simulink model "Test_anode_system"  (R2023a)
settings: Solver=VariableStepAuto  StartTime=0.0  StopTime=100  RelTol=1e-3
libraries: nesl_utility x13, fl_lib x8
settings Model: Creator=debjani.ghosh  LastModifiedBy=debjani.ghosh

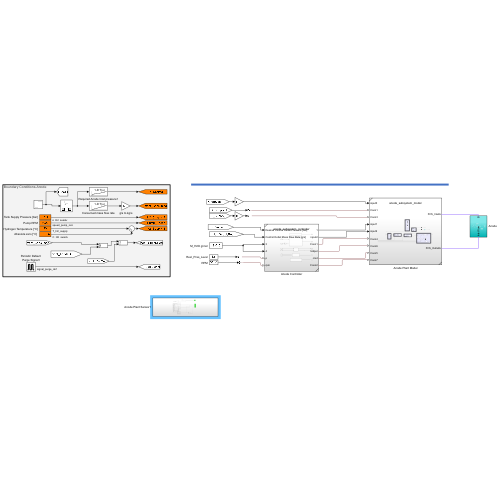
[thumbnail: Simulink's stored preview of the top-level diagram]
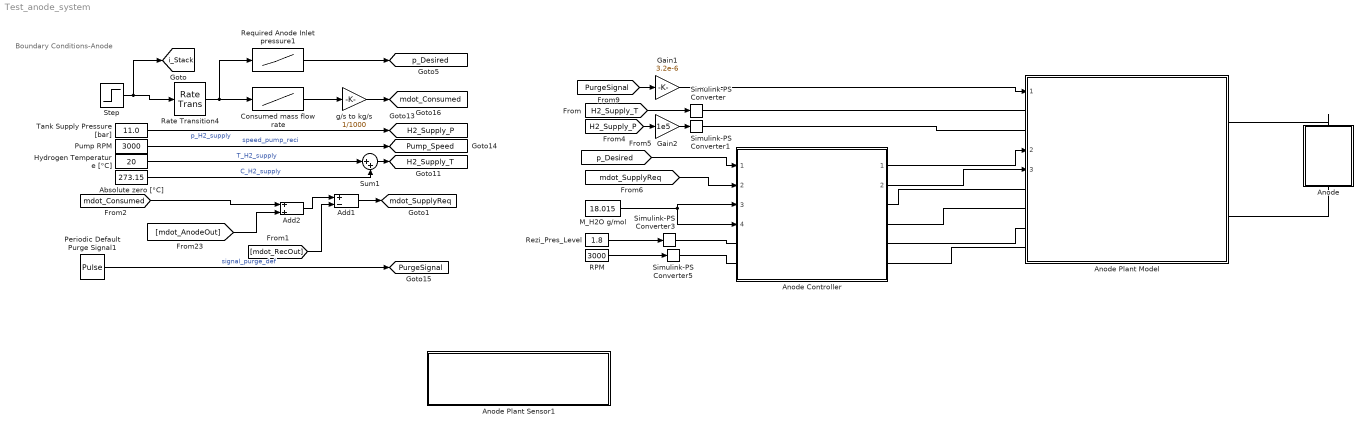
== system Test_anode_system ==
  note: Boundary Conditions-Anode
  "Absolute zero [°C] " : Constant  Value=273.15
  Add1 : Sum  Inputs=+-
  Add2 : Sum
  Anode : Subsystem  Tag=PublishSubsystem
  Anode Controller : Subsystem  ReferencedSubsystem=anode_subsystem_controller
  Anode Plant Model : Subsystem  ReferencedSubsystem=anode_subsystem_model
      settings: PortSchema="{\"entries\":[{\"content\":{\"sides\":[{\"content\":{\"connectorIds\":[\"In1\",\"LConn1\",\"LConn2\",\"In2\",\"In3\",\"LConn3\",\"LConn4\",\"LConn5\",\"LConn6\"]},\"type\":\"ConnectorPlacement.EquallySpacedRectSide\",\"uuid\":\"6d276737-1cfb-43f0-89a6-ca57f89f04f9\"},{\"content\":{\"connectorIds\":[\"RConn1\",\"RConn2\"],\"side\":\"RIGHT\"},\"type\":\"ConnectorPlacement.EquallySpacedRectSide\",\"uuid\":\"f7ce7b2b-f458-4a7d-a84b-f12d4a9a3d73\"},{\"content\":{\"side\":\"TOP\"},\"type\":\"ConnectorPlacement.EquallySpacedRectSide\",\"uuid\":\"f2759a84-f209-4626-aa5e-b52256180764\"}]},\"type\":\"ConnectorPlacement.EquallySpacedConnector\",\"uuid\":\"a55dce8e-c3c8-40fa-9a6a-dcd78737938e\"}],\"packageUris\":[\"http://schema.mathworks.com/mf0/Connector/R2020b\"],\"version\":\"1.0\"}"
  Anode Plant Sensor1 : Subsystem
  Consumed mass flow rate : Lookup_n-D  NumberOfTableDimensions=1  BreakpointsForDimension1=[0;20;100;200;300;400;500;600]  Table=[0;0.1;0.5;1;1.5;2;2.5;3]  InternalRulePriority=Speed  RndMeth=Simplest
  Gain1 : Gain  Gain=3.2e-6
  Gain2 : Gain  Gain=1e5
  Hydrogen Temperature [°C] : Constant  Value=20
  M_H2O g/mol : Constant  Value=18.015
  Periodic Default Purge Signal1 : DiscretePulseGenerator  PulseType=Time based  Period=3  PulseWidth=5
  Pump RPM : Constant  Value=3000
  RPM : Constant  Value=3000
  Rate Transition4 : RateTransition
  Required Anode Inlet pressure1 : Lookup_n-D  NumberOfTableDimensions=1  BreakpointsForDimension1=[0;20;100;200;300;400;500;600]  Table=[1;1.4;1.6;1.7;1.8;2;2.3;2.6]  InternalRulePriority=Speed  RndMeth=Simplest
  Rezi_Pres_Level : Constant  Value=1.8
  Simulink-PS Converter : nesl_utility/Simulink-PS Converter  PhysicalDomain=network_engine_domain  SubClassName=ps_input  LeftPortType=input  RightPortType=output  PseudoPeriodic=off  Frequencies=[]  NoiseDistribution=none  NoiseParameters=[]  Unit=K  AffineConversion=off  FilteringAndDerivatives=provide  SimscapeFilterOrder=1  InputFilterTimeConstant=0.001  UdotUserProvided=0
  Simulink-PS Converter1 : nesl_utility/Simulink-PS Converter  PhysicalDomain=network_engine_domain  SubClassName=ps_input  LeftPortType=input  RightPortType=output  PseudoPeriodic=off  Frequencies=[]  NoiseDistribution=none  NoiseParameters=[]  Unit=Pa  AffineConversion=off  FilteringAndDerivatives=provide  SimscapeFilterOrder=1  InputFilterTimeConstant=0.001  UdotUserProvided=0
  Simulink-PS Converter3 : nesl_utility/Simulink-PS Converter  PhysicalDomain=network_engine_domain  SubClassName=ps_input  LeftPortType=input  RightPortType=output  PseudoPeriodic=off  Frequencies=[]  NoiseDistribution=none  NoiseParameters=[]  Unit=1  AffineConversion=off  FilteringAndDerivatives=provide  SimscapeFilterOrder=1  InputFilterTimeConstant=0.001  UdotUserProvided=0
  Simulink-PS Converter5 : nesl_utility/Simulink-PS Converter  PhysicalDomain=network_engine_domain  SubClassName=ps_input  LeftPortType=input  RightPortType=output  PseudoPeriodic=off  Frequencies=[]  NoiseDistribution=none  NoiseParameters=[]  Unit=1  AffineConversion=off  FilteringAndDerivatives=provide  SimscapeFilterOrder=1  InputFilterTimeConstant=0.001  UdotUserProvided=0
  Step : Step  Time=50  Before=200  After=400  SampleTime=0
  Sum1 : Sum  Inputs=|++
  Tank Supply Pressure [bar] : Constant  Value=11.0
  g/s to kg/s : Gain  Gain=1/1000
  tag scope: H2_Supply_P=global, H2_Supply_T=global, Pump_Speed=global, PurgeSignal=global, i_Stack=global, mdot_Consumed=global, mdot_SupplyReq=global, p_Desired=global
  wires:
  Sum1/1 -> [H2_Supply_T]
  Gain1/1 -> Anode Plant Model/1
  [p_Desired] -> Anode Controller/1
  g/s to kg/s/1 -> [mdot_Consumed]
  [H2_Supply_T] -> Simulink-PS Converter/1
  "Absolute zero [°C] "/1 -> Sum1/2  "C_H2_supply"
  RPM/1 -> Simulink-PS Converter5/1
  Rezi_Pres_Level/1 -> Simulink-PS Converter3/1
  Periodic Default Purge Signal1/1 -> [PurgeSignal]  "signal_purge_def"
  Consumed mass flow rate/1 -> g/s to kg/s/1
  [PurgeSignal] -> Gain1/1
  [mdot_SupplyReq] -> Anode Controller/2
  [H2_Supply_P] -> Gain2/1
  Anode Controller/1 -> Anode Plant Model/2
  Gain2/1 -> Simulink-PS Converter1/1
  M_H2O g/mol/1 -> Anode Controller/3, Anode Controller/4
  Pump RPM/1 -> [Pump_Speed]  "speed_pump_reci"
  Rate Transition4/1 -> Required Anode Inlet pressure1/1, Consumed mass flow rate/1
  Required Anode Inlet pressure1/1 -> [p_Desired]
  Anode Controller/2 -> Anode Plant Model/3
  Tank Supply Pressure [bar]/1 -> [H2_Supply_P]  "p_H2_supply"
  Hydrogen Temperature [°C]/1 -> Sum1/1  "T_H2_supply"
  Step/1 -> [i_Stack], Rate Transition4/1
  [mdot_AnodeOut] -> Add2/2
  Add2/1 -> Add1/1
  [mdot_Consumed] -> Add2/1
  Add1/1 -> [mdot_SupplyReq]
  [mdot_RecOut] -> Add1/2
  connections:
  Simulink-PS Converter/RConn1 -- Anode Plant Model/LConn1
  Anode Plant Model/LConn6 -- Anode Controller/RConn4
  Anode Plant Model/LConn2 -- Simulink-PS Converter1/RConn1
  Anode Controller/RConn3 -- Anode Plant Model/LConn5
  Anode Controller/LConn1 -- Simulink-PS Converter3/RConn1
  Anode Controller/RConn2 -- Anode Plant Model/LConn4
  Anode Controller/RConn1 -- Anode Plant Model/LConn3
  Simulink-PS Converter5/RConn1 -- Anode Controller/LConn2
  Anode/LConn1 -- Anode Plant Model/RConn1
  Anode/RConn1 -- Anode Plant Model/RConn2

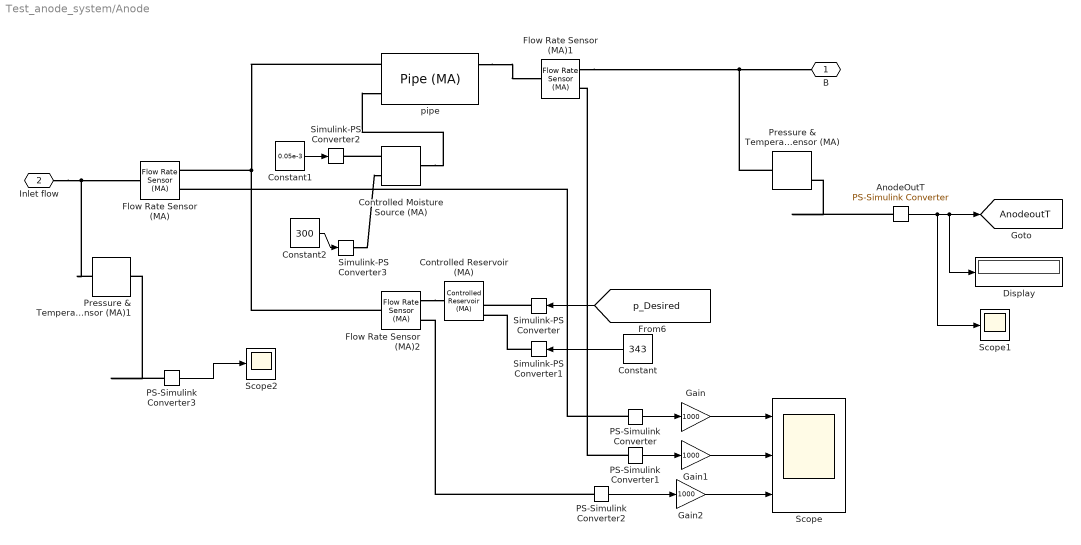
== system Test_anode_system/Anode ==
  AnodeOutT : nesl_utility/PS-Simulink Converter  PhysicalDomain=network_engine_domain  SubClassName=ps_output  LeftPortType=input  RightPortType=output  PseudoPeriodic=off  Frequencies=[]  VectorFormat=inherit  Unit=inherit  AffineConversion=off
  Constant : Constant  Value=343
  Constant1 : Constant  Value=0.05e-3
  Constant2 : Constant  Value=300
  Controlled Moisture Source (MA) : fl_lib/Moist Air/Sources/Moisture & Trace Gas Sources/Controlled Moisture Source (MA)  moisture_source_spec=foundation.enum.moisture_source_spec.vapor  Phi_S_specify=off  Phi_S_priority=None  Phi_S=0 kW  Phi_S_nominal_specify=off  Phi_S_nominal_unit=kW  Phi_S_nominal_value=1  mdot_w_S_specify=off  mdot_w_S_priority=None  mdot_w_S=0 kg/s  mdot_w_S_nominal_specify=off  mdot_w_S_nominal_unit=kg/s  mdot_w_S_nominal_value=1
      settings: InternalSimscapePortConfiguration="{\"Bottom\":[],\"Left\":[{\"id\":\"S\",\"label\":\"S\",\"type\":\"foundation.moist_air.moist_air_source\"}],\"Right\":[{\"id\":\"M\",\"label\":\"M\",\"type\":\"input\"},{\"id\":\"T\",\"label\":\"T\",\"type\":\"input\"}],\"Top\":[]}"
  Controlled Reservoir (MA) : fl_lib/Moist Air/Elements/Controlled Reservoir (MA)  moisture_spec=foundation.enum.moistureSpec.RelativeHumidity  trace_gas_spec=foundation.enum.trace_gas_spec.mass_fraction  RH_ws=1  area_A=0.01 m^2  input_error_spec=foundation.enum.input_range_error.warn
      settings: InternalSimscapePortConfiguration="{\"Bottom\":[],\"Left\":[{\"id\":\"A\",\"label\":\"A\",\"type\":\"foundation.moist_air.moist_air\"}],\"Right\":[{\"id\":\"T\",\"label\":\"T\",\"type\":\"input\"},{\"id\":\"P\",\"label\":\"P\",\"type\":\"input\"},{\"id\":\"W\",\"label\":\"W\",\"type\":\"input\"},{\"id\":\"G\",\"label\":\"G\",\"type\":\"input\"}],\"Top\":[]}"
  Display : Display
  Flow Rate Sensor (MA) : fl_lib/Moist Air/Sensors/Flow Rate Sensor (MA)  mass_flow_measure=true  volumetric_flow_measure=false  volumetric_flow_conditions=foundation.enum.volumetric_flow_conditions.actual  p_std=0.101325 MPa  T_std=20 degC  RH_std=0.65  energy_flow_measure=false  vapor_flow_measure=false  gas_flow_measure=false
      settings: InternalSimscapePortConfiguration="{\"Bottom\":[],\"Left\":[{\"id\":\"A\",\"label\":\"A\",\"type\":\"foundation.moist_air.moist_air\"}],\"Right\":[{\"id\":\"B\",\"label\":\"B\",\"type\":\"foundation.moist_air.moist_air\"},{\"id\":\"M\",\"label\":\"M\",\"type\":\"output\"}],\"Top\":[]}"
  Flow Rate Sensor (MA)1 : fl_lib/Moist Air/Sensors/Flow Rate Sensor (MA)  mass_flow_measure=true  volumetric_flow_measure=false  volumetric_flow_conditions=foundation.enum.volumetric_flow_conditions.actual  p_std=0.101325 MPa  T_std=20 degC  RH_std=0.65  energy_flow_measure=false  vapor_flow_measure=false  gas_flow_measure=false
      settings: InternalSimscapePortConfiguration="{\"Bottom\":[],\"Left\":[{\"id\":\"A\",\"label\":\"A\",\"type\":\"foundation.moist_air.moist_air\"}],\"Right\":[{\"id\":\"B\",\"label\":\"B\",\"type\":\"foundation.moist_air.moist_air\"},{\"id\":\"M\",\"label\":\"M\",\"type\":\"output\"}],\"Top\":[]}"
  Flow Rate Sensor (MA)2 : fl_lib/Moist Air/Sensors/Flow Rate Sensor (MA)  mass_flow_measure=true  volumetric_flow_measure=false  volumetric_flow_conditions=foundation.enum.volumetric_flow_conditions.actual  p_std=0.101325 MPa  T_std=20 degC  RH_std=0.65  energy_flow_measure=false  vapor_flow_measure=false  gas_flow_measure=false
      settings: InternalSimscapePortConfiguration="{\"Bottom\":[],\"Left\":[{\"id\":\"A\",\"label\":\"A\",\"type\":\"foundation.moist_air.moist_air\"}],\"Right\":[{\"id\":\"B\",\"label\":\"B\",\"type\":\"foundation.moist_air.moist_air\"},{\"id\":\"M\",\"label\":\"M\",\"type\":\"output\"}],\"Top\":[]}"
  Gain : Gain  Gain=1000
  Gain1 : Gain  Gain=1000
  Gain2 : Gain  Gain=1000
  PS-Simulink Converter{,1..3} (4 alike) : nesl_utility/PS-Simulink Converter  PhysicalDomain=network_engine_domain  SubClassName=ps_output  LeftPortType=input  RightPortType=output  PseudoPeriodic=off  Frequencies=[]  VectorFormat=inherit  Unit=inherit  AffineConversion=off
  Pressure & Temperature Sensor (MA) : fl_lib/Moist Air/Sensors/Pressure & Temperature Sensor (MA)  reference=foundation.enum.MeasurementReference.absolute  pressure=true  pressure_spec=foundation.enum.PressureMeasementSpec.Absolute  temperature=true
      settings: InternalSimscapePortConfiguration="{\"Bottom\":[{\"id\":\"T\",\"label\":\"T\",\"type\":\"output\"}],\"Left\":[{\"id\":\"A\",\"label\":\"A\",\"type\":\"foundation.moist_air.moist_air\"}],\"Right\":[{\"id\":\"Pa\",\"label\":\"Pa\",\"type\":\"output\"}],\"Top\":[]}"
  Pressure & Temperature Sensor (MA)1 : fl_lib/Moist Air/Sensors/Pressure & Temperature Sensor (MA)  reference=foundation.enum.MeasurementReference.absolute  pressure=false  pressure_spec=foundation.enum.PressureMeasementSpec.Absolute  temperature=true
      settings: InternalSimscapePortConfiguration="{\"Bottom\":[{\"id\":\"T\",\"label\":\"T\",\"type\":\"output\"}],\"Left\":[{\"id\":\"A\",\"label\":\"A\",\"type\":\"foundation.moist_air.moist_air\"}],\"Right\":[],\"Top\":[]}"
  Scope : Scope  NumInputPorts=3
  Scope1 : Scope
  Scope2 : Scope
  Simulink-PS Converter : nesl_utility/Simulink-PS Converter  PhysicalDomain=network_engine_domain  SubClassName=ps_input  LeftPortType=input  RightPortType=output  PseudoPeriodic=off  Frequencies=[]  NoiseDistribution=none  NoiseParameters=[]  Unit=bar  AffineConversion=off  FilteringAndDerivatives=provide  SimscapeFilterOrder=1  InputFilterTimeConstant=0.001  UdotUserProvided=0
  Simulink-PS Converter1 : nesl_utility/Simulink-PS Converter  PhysicalDomain=network_engine_domain  SubClassName=ps_input  LeftPortType=input  RightPortType=output  PseudoPeriodic=off  Frequencies=[]  NoiseDistribution=none  NoiseParameters=[]  Unit=K  AffineConversion=off  FilteringAndDerivatives=provide  SimscapeFilterOrder=1  InputFilterTimeConstant=0.001  UdotUserProvided=0
  Simulink-PS Converter2 : nesl_utility/Simulink-PS Converter  PhysicalDomain=network_engine_domain  SubClassName=ps_input  LeftPortType=input  RightPortType=output  PseudoPeriodic=off  Frequencies=[]  NoiseDistribution=none  NoiseParameters=[]  Unit=1  AffineConversion=off  FilteringAndDerivatives=provide  SimscapeFilterOrder=1  InputFilterTimeConstant=0.001  UdotUserProvided=0
  Simulink-PS Converter3 : nesl_utility/Simulink-PS Converter  PhysicalDomain=network_engine_domain  SubClassName=ps_input  LeftPortType=input  RightPortType=output  PseudoPeriodic=off  Frequencies=[]  NoiseDistribution=none  NoiseParameters=[]  Unit=1  AffineConversion=off  FilteringAndDerivatives=provide  SimscapeFilterOrder=1  InputFilterTimeConstant=0.001  UdotUserProvided=0
  pipe : fl_lib/Moist Air/Elements/Pipe (MA)  length=0.25 m  area=pi*0.05^2/4 m^2  Dh=0.05 m  length_add=0.1 m  roughness=15e-6 m  Re_lam=2000  Re_tur=4000  shape_factor=64  Nu_lam=3.66  wall_condensation=simscape.enum.onoff.off  RH_ws=1  time_constant=1e-3 s  moisture_trace_gas_source=foundation.enum.moisture_trace_gas_source.controlled  moisture_source_spec=foundation.enum.moisture_source_spec.vapor  moisture_mass_flow=0 kg/s  moisture_temperature_spec=foundation.enum.temperature_spec.atmospheric  moisture_temperature=293.15 K  trace_gas_mass_flow=0 kg/s  trace_gas_temperature_spec=foundation.enum.temperature_spec.atmospheric  trace_gas_temperature=293.15 K  p_I_specify=on  p_I_priority=High  p_I=env_p MPa  p_I_nominal_specify=off  p_I_nominal_unit=MPa  p_I_nominal_value=1  T_I_specify=on  T_I_priority=High  T_I=env_T degC  T_I_nominal_specify=off  T_I_nominal_unit=K  T_I_nominal_value=1  RH_I_specify=off  RH_I_priority=High  RH_I=0  RH_I_nominal_specify=off  RH_I_nominal_unit=1  RH_I_nominal_value=1  x_w_I_specify=off  x_w_I_priority=None  x_w_I=0  x_w_I_nominal_specify=off  x_w_I_nominal_unit=1  x_w_I_nominal_value=1  y_w_I_specify=off  y_w_I_priority=None  y_w_I=0  y_w_I_nominal_specify=off  y_w_I_nominal_unit=1  y_w_I_nominal_value=1  HR_I_specify=off  HR_I_priority=None  HR_I=0  HR_I_nominal_specify=off  HR_I_nominal_unit=1  HR_I_nominal_value=1  x_g_I_specify=on  x_g_I_priority=None  x_g_I=0  x_g_I_nominal_specify=off  x_g_I_nominal_unit=1  x_g_I_nominal_value=1  y_g_I_specify=on  y_g_I_priority=High  y_g_I=tank_yH2  y_g_I_nominal_specify=off  y_g_I_nominal_unit=1  y_g_I_nominal_value=1
      settings: InternalSimscapePortConfiguration="{\"Bottom\":[],\"Left\":[{\"id\":\"A\",\"label\":\"A\",\"type\":\"foundation.moist_air.moist_air\"},{\"id\":\"H\",\"label\":\"H\",\"type\":\"foundation.thermal.thermal\"},{\"id\":\"S\",\"label\":\"S\",\"type\":\"foundation.moist_air.moist_air_source\"}],\"Right\":[{\"id\":\"B\",\"label\":\"B\",\"type\":\"foundation.moist_air.moist_air\"},{\"id\":\"W\",\"label\":\"W\",\"type\":\"output\"},{\"id\":\"F\",\"label\":\"F\",\"type\":\"output\"}],\"Top\":[]}"
  B : PMIOPort  Side=Left
  Inlet flow : PMIOPort  Port=2  Side=Right
  tag scope: AnodeoutT=global
  wires:
  [p_Desired] -> Simulink-PS Converter/1
  Constant/1 -> Simulink-PS Converter1/1
  AnodeOutT/1 -> Scope1/1, Display/1, [AnodeoutT]
  PS-Simulink Converter/1 -> Gain/1
  PS-Simulink Converter1/1 -> Gain1/1
  PS-Simulink Converter2/1 -> Gain2/1
  Gain2/1 -> Scope/3
  Gain1/1 -> Scope/2
  Gain/1 -> Scope/1
  PS-Simulink Converter3/1 -> Scope2/1
  Constant1/1 -> Simulink-PS Converter2/1
  Constant2/1 -> Simulink-PS Converter3/1
  connections:
  Inlet flow/RConn1 -- Pressure & Temperature Sensor (MA)1/LConn1 -- Flow Rate Sensor (MA)/LConn1
  pipe/LConn1 -- Flow Rate Sensor (MA)2/LConn1 -- Flow Rate Sensor (MA)/RConn1
  Simulink-PS Converter/RConn1 -- Controlled Reservoir (MA)/RConn2
  Simulink-PS Converter1/RConn1 -- Controlled Reservoir (MA)/RConn1
  Flow Rate Sensor (MA)1/RConn1 -- Pressure & Temperature Sensor (MA)/LConn1 -- B/RConn1
  AnodeOutT/LConn1 -- Pressure & Temperature Sensor (MA)/RConn2
  pipe/RConn1 -- Flow Rate Sensor (MA)1/LConn1
  Flow Rate Sensor (MA)2/RConn1 -- Controlled Reservoir (MA)/LConn1
  PS-Simulink Converter2/LConn1 -- Flow Rate Sensor (MA)2/RConn2
  PS-Simulink Converter1/LConn1 -- Flow Rate Sensor (MA)1/RConn2
  PS-Simulink Converter/LConn1 -- Flow Rate Sensor (MA)/RConn2
  PS-Simulink Converter3/LConn1 -- Pressure & Temperature Sensor (MA)1/RConn1
  Controlled Moisture Source (MA)/RConn1 -- Simulink-PS Converter2/RConn1
  Controlled Moisture Source (MA)/LConn1 -- pipe/LConn3
  Simulink-PS Converter3/RConn1 -- Controlled Moisture Source (MA)/RConn2

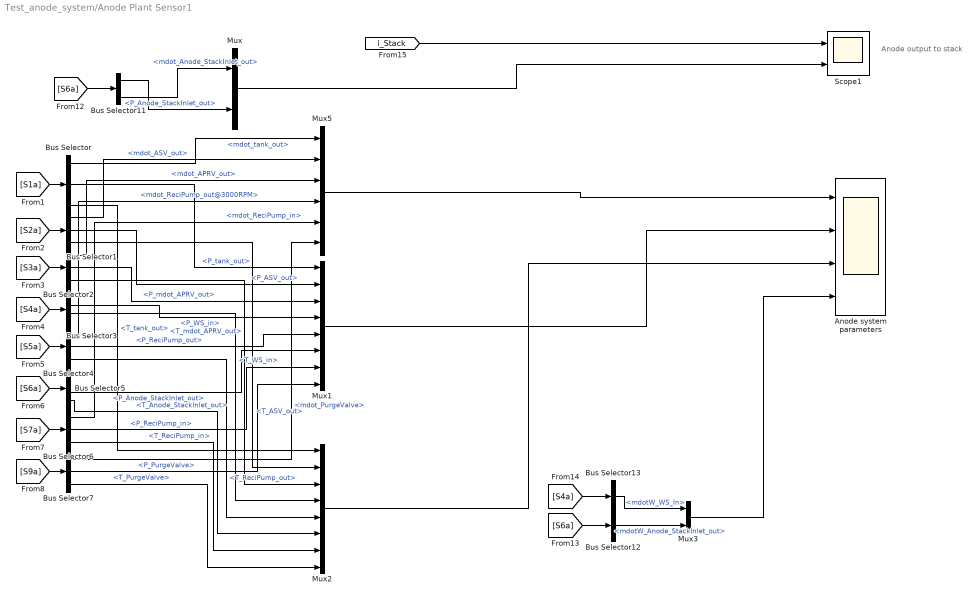
== system Test_anode_system/Anode Plant Sensor1 ==
  note: Anode output to stack
  Anode system parameters : Scope  NumInputPorts=4
  Bus Selector : BusSelector  OutputSignals=mdot_tank_out,P_tank_out,T_tank_out
  Bus Selector1 : BusSelector  OutputSignals=mdot_ASV_out,P_ASV_out,T_ASV_out
  Bus Selector11 : BusSelector  OutputSignals=P_Anode_StackInlet_out,mdot_Anode_StackInlet_out
  Bus Selector12 : BusSelector  OutputSignals=mdotW_Anode_StackInlet_out
  Bus Selector13 : BusSelector  OutputSignals=mdotW_WS_In
  Bus Selector2 : BusSelector  OutputSignals=mdot_APRV_out,P_mdot_APRV_out,T_mdot_APRV_out
  Bus Selector3 : BusSelector  OutputSignals=mdot_WS_in,P_WS_in,T_WS_in,mdotW_WS_In
  Bus Selector4 : BusSelector  OutputSignals=mdot_ReciPump_out@3000RPM,P_ReciPump_out,T_ReciPump_out
  Bus Selector5 : BusSelector  OutputSignals=mdot_Anode_StackInlet_out,mdotW_Anode_StackInlet_out,P_Anode_StackInlet_out,T_Anode_StackInlet_out
  Bus Selector6 : BusSelector  OutputSignals=mdot_ReciPump_in,P_ReciPump_in,T_ReciPump_in
  Bus Selector7 : BusSelector  OutputSignals=mdot_PurgeValve,P_PurgeValve,T_PurgeValve
  Mux : Mux  Inputs=2
  Mux1 : Mux  Inputs=8
  Mux2 : Mux  Inputs=8
  Mux3 : Mux  Inputs=2
  Mux5 : Mux  Inputs=6
  Scope1 : Scope  NumInputPorts=2
  wires:
  Bus Selector7/3 -> Mux2/8  "<T_PurgeValve>"
  Bus Selector6/3 -> Mux2/7  "<T_ReciPump_in>"
  Bus Selector5/4 -> Mux2/6  "<T_Anode_StackInlet_out>"
  Bus Selector4/3 -> Mux2/5  "<T_ReciPump_out>"
  Bus Selector3/3 -> Mux2/4  "<T_WS_in>"
  Bus Selector2/3 -> Mux2/3  "<T_mdot_APRV_out>"
  Bus Selector1/3 -> Mux2/2  "<T_ASV_out>"
  Bus Selector/3 -> Mux2/1  "<T_tank_out>"
  Bus Selector3/2 -> Mux1/4  "<P_WS_in>"
  Bus Selector4/2 -> Mux1/5  "<P_ReciPump_out>"
  Bus Selector2/2 -> Mux1/3  "<P_mdot_APRV_out>"
  Bus Selector1/2 -> Mux1/2  "<P_ASV_out>"
  Bus Selector/2 -> Mux1/1  "<P_tank_out>"
  Bus Selector6/2 -> Mux1/7  "<P_ReciPump_in>"
  Bus Selector7/2 -> Mux1/8  "<P_PurgeValve>"
  [S9a] -> Bus Selector7/1
  [S7a] -> Bus Selector6/1
  [S6a] -> Bus Selector5/1
  [S5a] -> Bus Selector4/1
  [S4a] -> Bus Selector3/1
  [S3a] -> Bus Selector2/1
  [S2a] -> Bus Selector1/1
  [S1a] -> Bus Selector/1
  Bus Selector5/3 -> Mux1/6  "<P_Anode_StackInlet_out>"
  [S6a] -> Bus Selector11/1
  Bus Selector11/2 -> Mux/1  "<mdot_Anode_StackInlet_out>"
  [S6a] -> Bus Selector12/1
  Bus Selector12/1 -> Mux3/2  "<mdotW_Anode_StackInlet_out>"
  [S4a] -> Bus Selector13/1
  Bus Selector13/1 -> Mux3/1  "<mdotW_WS_In>"
  Bus Selector11/1 -> Mux/2  "<P_Anode_StackInlet_out>"
  Bus Selector/1 -> Mux5/1  "<mdot_tank_out>"
  Bus Selector1/1 -> Mux5/2  "<mdot_ASV_out>"
  Bus Selector2/1 -> Mux5/3  "<mdot_APRV_out>"
  Bus Selector4/1 -> Mux5/4  "<mdot_ReciPump_out@3000RPM>"
  Bus Selector6/1 -> Mux5/5  "<mdot_ReciPump_in>"
  Bus Selector7/1 -> Mux5/6  "<mdot_PurgeValve>"
  Mux/1 -> Scope1/2
  [i_Stack] -> Scope1/1
  Mux5/1 -> Anode system parameters/1
  Mux1/1 -> Anode system parameters/2
  Mux2/1 -> Anode system parameters/3
  Mux3/1 -> Anode system parameters/4
